simulink model "Copy_of_Rocky"  (R2022a)
settings: Solver=VariableStepAuto  StartTime=0.0  StopTime=5  RelTol=1e-3
undefined symbols (not defined in the file): a, b, Ci, g, JiCp, Jp, Ki, Kp, l
settings Model: Creator=atan  LastModifiedBy=mluser
settings SolverCC: AlgebraicLoopSolver=TrustRegion
settings DebuggingCC: UnconnectedInputMsg=warning  UnconnectedOutputMsg=warning  UnconnectedLineMsg=warning  SFMachineParentedDataDiag=warning
settings RTWCC: DLArmComputeVersion=19.05

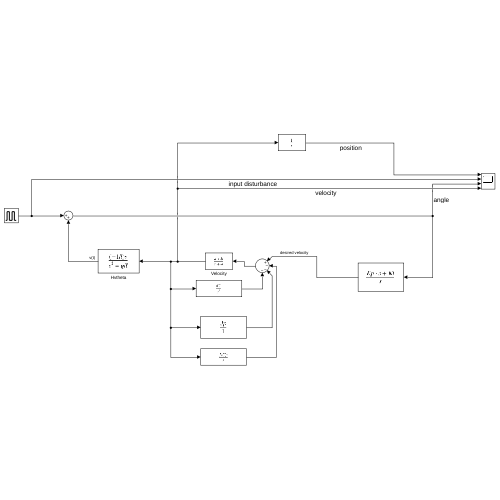
[thumbnail: Simulink's stored preview of the top-level diagram]
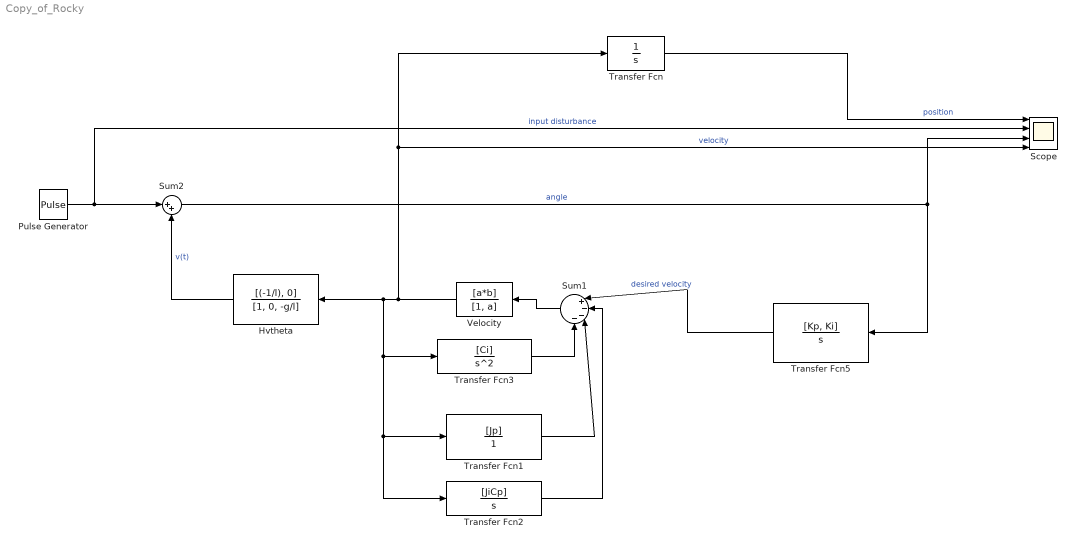
== system Copy_of_Rocky ==
  Hvtheta : TransferFcn  Numerator=[(-1/l), 0]  Denominator=[1, 0, -g/l]
  Pulse Generator : DiscretePulseGenerator  PulseType=Time based  Period=10  PulseWidth=5
  Scope : Scope  NumInputPorts=4
  Sum1 : Sum  Inputs=|+---
  Sum2 : Sum  Inputs=|++
  Transfer Fcn : TransferFcn  Denominator=[ 1 0]
  Transfer Fcn1 : TransferFcn  Numerator=[Jp]  Denominator=[1]
  Transfer Fcn2 : TransferFcn  Numerator=[JiCp]  Denominator=[1 , 0]
  Transfer Fcn3 : TransferFcn  Numerator=[Ci]  Denominator=[1 , 0, 0]
  Transfer Fcn5 : TransferFcn  Numerator=[Kp, Ki]  Denominator=[1 0]
  Velocity : TransferFcn  Numerator=[a*b]  Denominator=[1, a]
  wires:
  Velocity/1 -> Transfer Fcn2/1, Transfer Fcn1/1, Transfer Fcn3/1, Hvtheta/1, Transfer Fcn/1, Scope/4  "velocity"
  Sum1/1 -> Velocity/1
  Transfer Fcn1/1 -> Sum1/3
  Transfer Fcn2/1 -> Sum1/2
  Transfer Fcn5/1 -> Sum1/1  "desired velocity"
  Hvtheta/1 -> Sum2/2  "v(t)"
  Sum2/1 -> Scope/3, Transfer Fcn5/1  "angle"
  Pulse Generator/1 -> Scope/2, Sum2/1  "input disturbance"
  Transfer Fcn/1 -> Scope/1  "position"
  Transfer Fcn3/1 -> Sum1/4
